simulink model "Appl_DrRestMode_CtrlModel"  (R2018b)
settings: configuration reference "CodeConfig_10_ms" (kept outside this file)
undefined symbols (not defined in the file): D_ClickNapBackPosi, D_ClickNapLengthPosi, D_DRMEM_SPEED_5, D_SoftDistanceDrLegnth, FALSE, TRUE
libraries: DareLib x81, simulink x1
(part 1 of 2)
settings Model: Creator=Administrator  LastModifiedBy=Administrator
settings ConfigSetRef: SourceLocation=Base Workspace

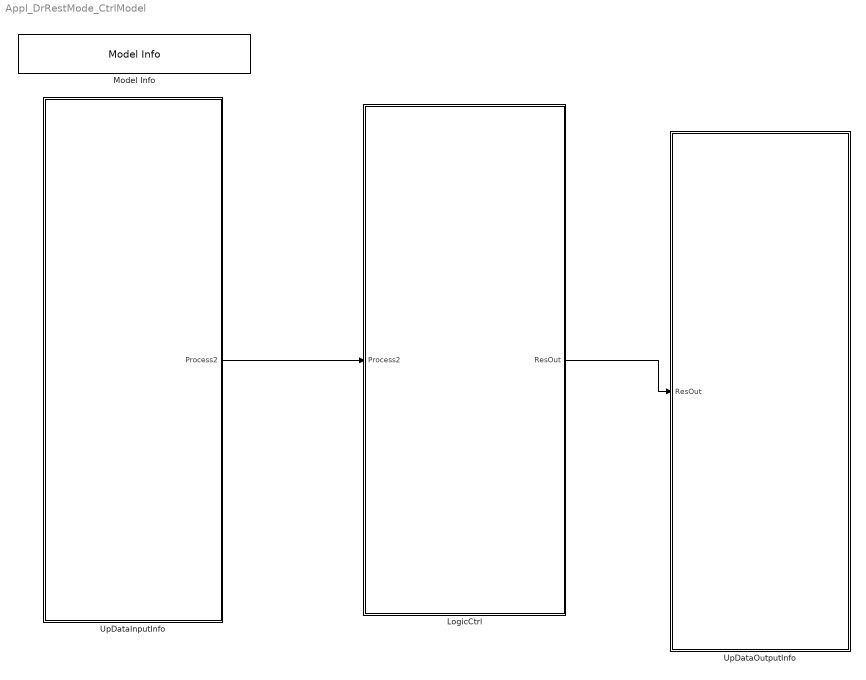
== system Appl_DrRestMode_CtrlModel ==
  LogicCtrl : Subsystem  Priority=2  TreatAsAtomicUnit=on
      settings: RTWSystemCode=Nonreusable function  RTWFcnNameOpts=Use subsystem name
  Model Info : simulink/Model-Wide Utilities/Model Info  Frame=on  DisplayStringWithTags=Version：%<ModelVersion>  HorizontalTextAlignment=Center  LeftAlignmentValue=0.5
  UpDataInputInfo : Subsystem  Priority=1  TreatAsAtomicUnit=on
      settings: RTWSystemCode=Nonreusable function  RTWFcnNameOpts=Use subsystem name
  UpDataOutputInfo : Subsystem  Priority=3  TreatAsAtomicUnit=on
      settings: RTWSystemCode=Nonreusable function  RTWFcnNameOpts=Use subsystem name
  wires:
  LogicCtrl/1(ResOut) -> UpDataOutputInfo/1(ResOut)
  UpDataInputInfo/1(Process2) -> LogicCtrl/1(Process2)

== system Appl_DrRestMode_CtrlModel/LogicCtrl ==
  Process2 : Inport
  Bus Creator : BusCreator  Inputs=13
  Bus Selector : BusSelector  OutputSignals=Res_Stop_Flag.Stop_Flag,Res_Open_Flag.Open_Flag,Res_Close_Flag.Close_Flag,MotorFault_Flag,MassageFault_Flag,DrRestCAll_Ret,Process1.CallHallValue.CallHallVall_Height,Process1.CallHallValue.CallHallVall_Length,Process1.CallHallValue.CallHallVall_Back,Process1.CallHallValue.CallHallVall_Front,Process1.Rte_SignalBus1.DrRes_HeightHallPosi,Process1.Rte_SignalBus1.DrRes_LengthHallPosi,Process1.Rte_SignalBus1.DrRes_BackHallPosi,Process1.Rte_SignalBus1.DrRes_FrontHallPosi,Process1.Rte_SignalBus1.DrRes_AnyoneRelayFaultSts,Process1.Rte_SignalBus1.DrResl_ReCallPosi_Height,Process1.Rte_SignalBus1.DrResl_ReCallPosi_Length,Process1.Rte_SignalBus1.DrResl_ReCallPosi_Back,Process1.Rte_SignalBus1.DrResl_ReCallPosi_Front,Process1.Rte_SignalBus1.DrRes_CurrentMoveType
  ResCtrl : Subsystem  Description=小憩逻辑处理
      settings: AttributesFormatString=%<Description>
  ResOut : Outport
  wires:
  Process2/1 -> Bus Creator/13, Bus Selector/1  "Process2"
  Bus Creator/1 -> ResOut/1  "ResOut"
  ResCtrl/3(DSM_NapMode_FB) -> Bus Creator/3
  ResCtrl/2(DSM_MassageMode_Req) -> Bus Creator/2
  ResCtrl/4(ResCallPosi_Height) -> Bus Creator/4
  ResCtrl/1(DSM_MassageLevel_Req) -> Bus Creator/1
  ResCtrl/5(ResCallPosi_Length) -> Bus Creator/5
  ResCtrl/6(ResCallPosi_Front) -> Bus Creator/6
  ResCtrl/7(ResCallPosi_Back) -> Bus Creator/7
  ResCtrl/8(ResReCallPosi_Back) -> Bus Creator/8
  ResCtrl/9(ResReCallPosi_Front) -> Bus Creator/9
  ResCtrl/10(ResReCallPosi_Height) -> Bus Creator/10
  ResCtrl/11(ResReCallPosi_Length) -> Bus Creator/11
  ResCtrl/12(State_ResDeal) -> Bus Creator/12
  Bus Selector/1 -> ResCtrl/1(Stop_Flag)  "<Stop_Flag>"
  Bus Selector/2 -> ResCtrl/2(Open_Flag)  "<Open_Flag>"
  Bus Selector/3 -> ResCtrl/3(Close_Flag)  "<Close_Flag>"
  Bus Selector/4 -> ResCtrl/4(MotorFault_Flag)  "<MotorFault_Flag>"
  Bus Selector/5 -> ResCtrl/5(MassageFault_Flag)  "<MassageFault_Flag>"
  Bus Selector/6 -> ResCtrl/6(DrRestCAll_Ret)  "<DrRestCAll_Ret>"
  Bus Selector/7 -> ResCtrl/7(CallHallVall_Height)  "<CallHallVall_Height>"
  Bus Selector/8 -> ResCtrl/8(CallHallVall_Length)  "<CallHallVall_Length>"
  Bus Selector/9 -> ResCtrl/9(CallHallVall_Back)  "<CallHallVall_Back>"
  Bus Selector/10 -> ResCtrl/10(CallHallVall_Front)  "<CallHallVall_Front>"
  Bus Selector/11 -> ResCtrl/11(DrRes_HeightHallPosi)  "<DrRes_HeightHallPosi>"
  Bus Selector/12 -> ResCtrl/12(DrRes_LengthHallPosi)  "<DrRes_LengthHallPosi>"
  Bus Selector/13 -> ResCtrl/13(DrRes_BackHallPosi)  "<DrRes_BackHallPosi>"
  Bus Selector/14 -> ResCtrl/14(DrRes_FrontHallPosi)  "<DrRes_FrontHallPosi>"
  Bus Selector/15 -> ResCtrl/15(DrRes_AnyoneRelayFaultSts)  "<DrRes_AnyoneRelayFaultSts>"
  Bus Selector/16 -> ResCtrl/16(DrResl_ReCallPosi_Height)  "<DrResl_ReCallPosi_Height>"
  Bus Selector/17 -> ResCtrl/17(DrResl_ReCallPosi_Length)  "<DrResl_ReCallPosi_Length>"
  Bus Selector/18 -> ResCtrl/18(DrResl_ReCallPosi_Back)  "<DrResl_ReCallPosi_Back>"
  Bus Selector/19 -> ResCtrl/19(DrResl_ReCallPosi_Front)  "<DrResl_ReCallPosi_Front>"
  Bus Selector/20 -> ResCtrl/20(DrRes_CurrentMoveType)  "<DrRes_CurrentMoveType>"

== system Appl_DrRestMode_CtrlModel/UpDataInputInfo ==
  InputSignalProcess1 : Subsystem  Description=预处理1
      settings: AttributesFormatString=%<Description>  RTWSystemCode=Nonreusable function  RTWFcnNameOpts=Use subsystem name
  InputSignalProcess2 : Subsystem  Description=预处理2
      settings: AttributesFormatString=%<Description>  RTWSystemCode=Nonreusable function  RTWFcnNameOpts=Use subsystem name
  RTE : Subsystem  Description=接口自动生成  TreatAsAtomicUnit=on
      settings: AttributesFormatString=%<Description>  RTWSystemCode=Nonreusable function  RTWFcnNameOpts=Use subsystem name
  Process2 : Outport
  wires:
  RTE/1(RTE_Signal) -> InputSignalProcess1/1(Rte_SignalBus)
  InputSignalProcess1/1(Process1) -> InputSignalProcess2/1(Process1)
  InputSignalProcess2/1(Process2) -> Process2/1

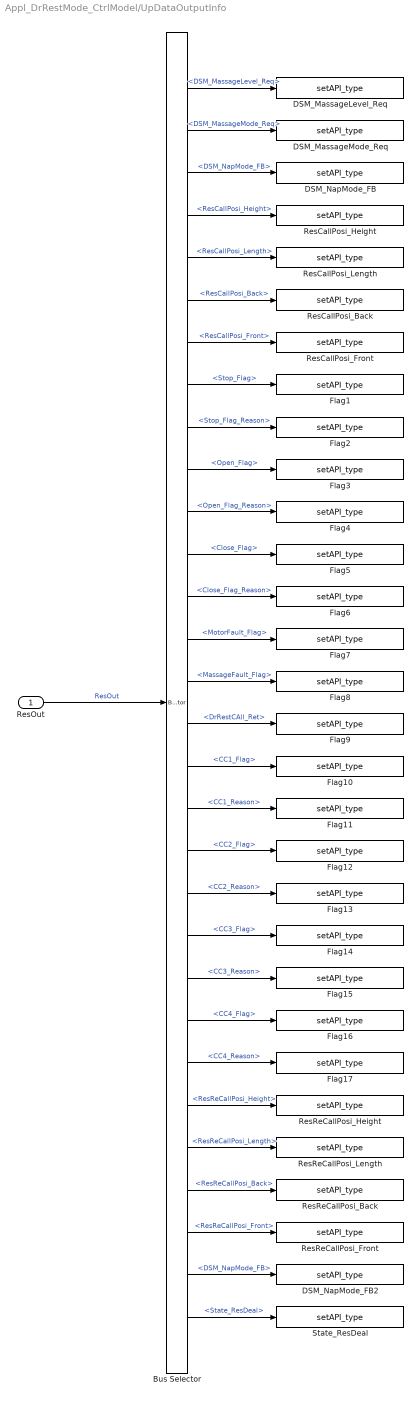
== system Appl_DrRestMode_CtrlModel/UpDataOutputInfo ==
  ResOut : Inport
  Bus Selector : BusSelector  OutputSignals=DSM_MassageLevel_Req,DSM_MassageMode_Req,DSM_NapMode_FB,ResCallPosi_Height,ResCallPosi_Length,ResCallPosi_Back,ResCallPosi_Front,Process2.Res_Stop_Flag.Stop_Flag,Process2.Res_Stop_Flag.Stop_Flag_Reason,Process2.Res_Open_Flag.Open_Flag,Process2.Res_Open_Flag.Open_Flag_Reason,Process2.Res_Close_Flag.Close_Flag,Process2.Res_Close_Flag.Close_Flag_Reason,Process2.MotorFault_Flag,Process2.MassageFault_Flag,Process2.DrRestCAll_Ret,Process2.Process1.CC1.CC1_Flag,Process2.Process1.CC1.CC1_Reason,Process2.Process1.CC2.CC2_Flag,Process2.Process1.CC2.CC2_Reason,Process2.Process1.CC3.CC3_Flag,Process2.Process1.CC3.CC3_Reason,Process2.Process1.CC4.CC4_Flag,Process2.Process1.CC4.CC4_Reason,ResReCallPosi_Height,ResReCallPosi_Length,ResReCallPosi_Back,ResReCallPosi_Front,DSM_NapMode_FB,State_ResDeal
  DSM_MassageLevel_Req : DareLib/Dare/setAPI_type  g_funcname=Rte_SetVfb_Res_MassageLevel_Req  g_param=""  g_type=uint8  g_size=-1
      settings: AttributesFormatString=%<g_funcname>  SourceProductName=Dare Library
  DSM_MassageMode_Req : DareLib/Dare/setAPI_type  g_funcname=Rte_SetVfb_Res_MassageMode_Req  g_param=""  g_type=uint8  g_size=-1
      settings: AttributesFormatString=%<g_funcname>  SourceProductName=Dare Library
  DSM_NapMode_FB : DareLib/Dare/setAPI_type  g_funcname=CanTx_0x3B2_DSM_NapMode_FB  g_param=""  g_type=uint8  g_size=-1
      settings: AttributesFormatString=%<g_funcname>  SourceProductName=Dare Library
  DSM_NapMode_FB2 : DareLib/Dare/setAPI_type  g_funcname=Rte_SetVfb_NapMode  g_param=""  g_type=uint8  g_size=-1
      settings: AttributesFormatString=%<g_funcname>  SourceProductName=Dare Library
  Flag1 : DareLib/Dare/setAPI_type  g_funcname=Rte_SetVfb_Debug_Res_Stop_Flag  g_param=""  g_type=uint8  g_size=-1
      settings: AttributesFormatString=%<g_funcname>  SourceProductName=Dare Library
  Flag10 : DareLib/Dare/setAPI_type  g_funcname=Rte_SetVfb_Debug_Res_CC1_Flag  g_param=""  g_type=uint8  g_size=-1
      settings: AttributesFormatString=%<g_funcname>  SourceProductName=Dare Library
  Flag11 : DareLib/Dare/setAPI_type  g_funcname=Rte_SetVfb_Debug_Res_CC1_Reason  g_param=""  g_type=uint8  g_size=-1
      settings: AttributesFormatString=%<g_funcname>  SourceProductName=Dare Library
  Flag12 : DareLib/Dare/setAPI_type  g_funcname=Rte_SetVfb_Debug_Res_CC2_Flag  g_param=""  g_type=uint8  g_size=-1
      settings: AttributesFormatString=%<g_funcname>  SourceProductName=Dare Library
  Flag13 : DareLib/Dare/setAPI_type  g_funcname=Rte_SetVfb_Debug_Res_CC2_Reason  g_param=""  g_type=uint8  g_size=-1
      settings: AttributesFormatString=%<g_funcname>  SourceProductName=Dare Library
  Flag14 : DareLib/Dare/setAPI_type  g_funcname=Rte_SetVfb_Debug_Res_CC3_Flag  g_param=""  g_type=uint8  g_size=-1
      settings: AttributesFormatString=%<g_funcname>  SourceProductName=Dare Library
  Flag15 : DareLib/Dare/setAPI_type  g_funcname=Rte_SetVfb_Debug_Res_CC3_Reason  g_param=""  g_type=uint8  g_size=-1
      settings: AttributesFormatString=%<g_funcname>  SourceProductName=Dare Library
  Flag16 : DareLib/Dare/setAPI_type  g_funcname=Rte_SetVfb_Debug_Res_CC4_Flag  g_param=""  g_type=uint8  g_size=-1
      settings: AttributesFormatString=%<g_funcname>  SourceProductName=Dare Library
  Flag17 : DareLib/Dare/setAPI_type  g_funcname=Rte_SetVfb_Debug_Res_CC4_Reason  g_param=""  g_type=uint8  g_size=-1
      settings: AttributesFormatString=%<g_funcname>  SourceProductName=Dare Library
  Flag2 : DareLib/Dare/setAPI_type  g_funcname=Rte_SetVfb_Debug_Res_Stop_Flag_Reason  g_param=""  g_type=uint8  g_size=-1
      settings: AttributesFormatString=%<g_funcname>  SourceProductName=Dare Library
  Flag3 : DareLib/Dare/setAPI_type  g_funcname=Rte_SetVfb_Debug_Res_Open_Flag  g_param=""  g_type=uint8  g_size=-1
      settings: AttributesFormatString=%<g_funcname>  SourceProductName=Dare Library
  Flag4 : DareLib/Dare/setAPI_type  g_funcname=Rte_SetVfb_Debug_Res_Open_Flag_Reason  g_param=""  g_type=uint8  g_size=-1
      settings: AttributesFormatString=%<g_funcname>  SourceProductName=Dare Library
  Flag5 : DareLib/Dare/setAPI_type  g_funcname=Rte_SetVfb_Debug_Res_Colse_Flag  g_param=""  g_type=uint8  g_size=-1
      settings: AttributesFormatString=%<g_funcname>  SourceProductName=Dare Library
  Flag6 : DareLib/Dare/setAPI_type  g_funcname=Rte_SetVfb_Debug_Res_Colse_Flag_Reason  g_param=""  g_type=uint8  g_size=-1
      settings: AttributesFormatString=%<g_funcname>  SourceProductName=Dare Library
  Flag7 : DareLib/Dare/setAPI_type  g_funcname=Rte_SetVfb_Debug_Res_MotroFault_Flag  g_param=""  g_type=uint8  g_size=-1
      settings: AttributesFormatString=%<g_funcname>  SourceProductName=Dare Library
  Flag8 : DareLib/Dare/setAPI_type  g_funcname=Rte_SetVfb_Debug_Res_MassageFault_Flag  g_param=""  g_type=uint8  g_size=-1
      settings: AttributesFormatString=%<g_funcname>  SourceProductName=Dare Library
  Flag9 : DareLib/Dare/setAPI_type  g_funcname=Rte_SetVfb_Debug_Res_DrRestCAllRet  g_param=""  g_type=uint8  g_size=-1
      settings: AttributesFormatString=%<g_funcname>  SourceProductName=Dare Library
  ResCallPosi_Back : DareLib/Dare/setAPI_type  g_funcname=Rte_SetVfb_DrResBackReqPosi  g_param=""  g_type=uint16  g_size=-1
      settings: AttributesFormatString=%<g_funcname>  SourceProductName=Dare Library
  ResCallPosi_Front : DareLib/Dare/setAPI_type  g_funcname=Rte_SetVfb_DrResFrontReqPosi  g_param=""  g_type=uint16  g_size=-1
      settings: AttributesFormatString=%<g_funcname>  SourceProductName=Dare Library
  ResCallPosi_Height : DareLib/Dare/setAPI_type  g_funcname=Rte_SetVfb_DrResHeightReqPosi  g_param=""  g_type=uint16  g_size=-1
      settings: AttributesFormatString=%<g_funcname>  SourceProductName=Dare Library
  ResCallPosi_Length : DareLib/Dare/setAPI_type  g_funcname=Rte_SetVfb_DrResLengthReqPosi  g_param=""  g_type=uint16  g_size=-1
      settings: AttributesFormatString=%<g_funcname>  SourceProductName=Dare Library
  ResReCallPosi_Back : DareLib/Dare/setAPI_type  g_funcname=Rte_SetVfb_DrResBackReCallPosi  g_param=""  g_type=uint16  g_size=-1
      settings: AttributesFormatString=%<g_funcname>  SourceProductName=Dare Library
  ResReCallPosi_Front : DareLib/Dare/setAPI_type  g_funcname=Rte_SetVfb_DrResFrontReCallPosi  g_param=""  g_type=uint16  g_size=-1
      settings: AttributesFormatString=%<g_funcname>  SourceProductName=Dare Library
  ResReCallPosi_Height : DareLib/Dare/setAPI_type  g_funcname=Rte_SetVfb_DrResHeightReCallPosi  g_param=""  g_type=uint16  g_size=-1
      settings: AttributesFormatString=%<g_funcname>  SourceProductName=Dare Library
  ResReCallPosi_Length : DareLib/Dare/setAPI_type  g_funcname=Rte_SetVfb_DrResLengthReCallPosi  g_param=""  g_type=uint16  g_size=-1
      settings: AttributesFormatString=%<g_funcname>  SourceProductName=Dare Library
  State_ResDeal : DareLib/Dare/setAPI_type  g_funcname=Rte_SetVfb_Debug_Res_State_ResDeal  g_param=""  g_type=uint8  g_size=-1
      settings: AttributesFormatString=%<g_funcname>  SourceProductName=Dare Library
  wires:
  ResOut/1 -> Bus Selector/1  "ResOut"
  Bus Selector/30 -> State_ResDeal/1  "<State_ResDeal>"
  Bus Selector/29 -> DSM_NapMode_FB2/1  "<DSM_NapMode_FB>"
  Bus Selector/28 -> ResReCallPosi_Front/1  "<ResReCallPosi_Front>"
  Bus Selector/27 -> ResReCallPosi_Back/1  "<ResReCallPosi_Back>"
  Bus Selector/26 -> ResReCallPosi_Length/1  "<ResReCallPosi_Length>"
  Bus Selector/25 -> ResReCallPosi_Height/1  "<ResReCallPosi_Height>"
  Bus Selector/24 -> Flag17/1  "<CC4_Reason>"
  Bus Selector/23 -> Flag16/1  "<CC4_Flag>"
  Bus Selector/22 -> Flag15/1  "<CC3_Reason>"
  Bus Selector/21 -> Flag14/1  "<CC3_Flag>"
  Bus Selector/20 -> Flag13/1  "<CC2_Reason>"
  Bus Selector/19 -> Flag12/1  "<CC2_Flag>"
  Bus Selector/18 -> Flag11/1  "<CC1_Reason>"
  Bus Selector/17 -> Flag10/1  "<CC1_Flag>"
  Bus Selector/16 -> Flag9/1  "<DrRestCAll_Ret>"
  Bus Selector/15 -> Flag8/1  "<MassageFault_Flag>"
  Bus Selector/14 -> Flag7/1  "<MotorFault_Flag>"
  Bus Selector/13 -> Flag6/1  "<Close_Flag_Reason>"
  Bus Selector/12 -> Flag5/1  "<Close_Flag>"
  Bus Selector/11 -> Flag4/1  "<Open_Flag_Reason>"
  Bus Selector/10 -> Flag3/1  "<Open_Flag>"
  Bus Selector/9 -> Flag2/1  "<Stop_Flag_Reason>"
  Bus Selector/8 -> Flag1/1  "<Stop_Flag>"
  Bus Selector/7 -> ResCallPosi_Front/1  "<ResCallPosi_Front>"
  Bus Selector/6 -> ResCallPosi_Back/1  "<ResCallPosi_Back>"
  Bus Selector/5 -> ResCallPosi_Length/1  "<ResCallPosi_Length>"
  Bus Selector/4 -> ResCallPosi_Height/1  "<ResCallPosi_Height>"
  Bus Selector/3 -> DSM_NapMode_FB/1  "<DSM_NapMode_FB>"
  Bus Selector/2 -> DSM_MassageMode_Req/1  "<DSM_MassageMode_Req>"
  Bus Selector/1 -> DSM_MassageLevel_Req/1  "<DSM_MassageLevel_Req>"

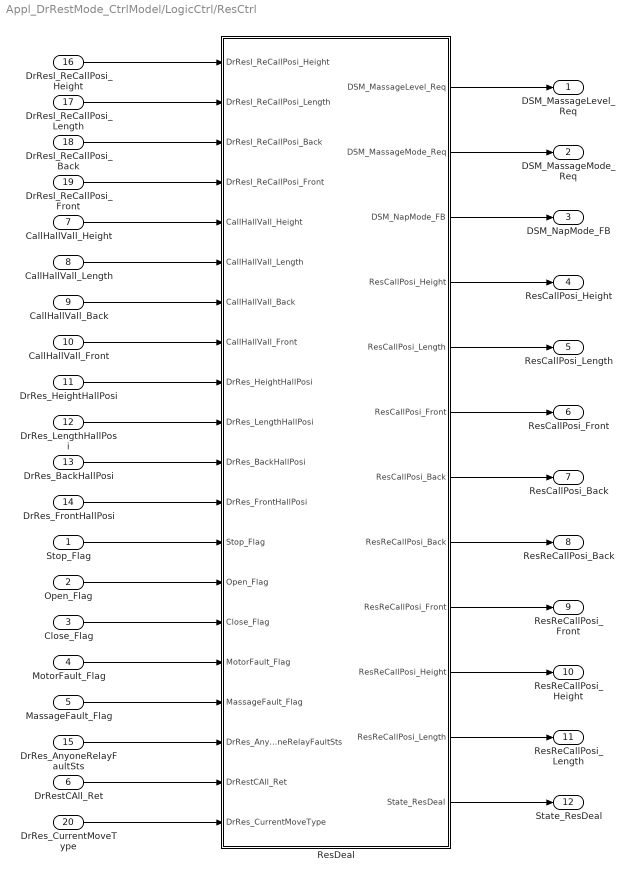
== system Appl_DrRestMode_CtrlModel/LogicCtrl/ResCtrl ==
  Stop_Flag : Inport
  Open_Flag : Inport  Port=2
  Close_Flag : Inport  Port=3
  MotorFault_Flag : Inport  Port=4
  MassageFault_Flag : Inport  Port=5
  DrRestCAll_Ret : Inport  Port=6
  CallHallVall_Height : Inport  Port=7
  CallHallVall_Length : Inport  Port=8
  CallHallVall_Back : Inport  Port=9
  CallHallVall_Front : Inport  Port=10
  DrRes_HeightHallPosi : Inport  Port=11
  DrRes_LengthHallPosi : Inport  Port=12
  DrRes_BackHallPosi : Inport  Port=13
  DrRes_FrontHallPosi : Inport  Port=14
  DrRes_AnyoneRelayFaultSts : Inport  Port=15
  DrResl_ReCallPosi_Height : Inport  Port=16
  DrResl_ReCallPosi_Length : Inport  Port=17
  DrResl_ReCallPosi_Back : Inport  Port=18
  DrResl_ReCallPosi_Front : Inport  Port=19
  DrRes_CurrentMoveType : Inport  Port=20
  ResDeal : Stateflow chart  TreatAsAtomicUnit=on
  DSM_MassageLevel_Req : Outport
  DSM_MassageMode_Req : Outport  Port=2
  DSM_NapMode_FB : Outport  Port=3
  ResCallPosi_Height : Outport  Port=4
  ResCallPosi_Length : Outport  Port=5
  ResCallPosi_Front : Outport  Port=6
  ResCallPosi_Back : Outport  Port=7
  ResReCallPosi_Back : Outport  Port=8
  ResReCallPosi_Front : Outport  Port=9
  ResReCallPosi_Height : Outport  Port=10
  ResReCallPosi_Length : Outport  Port=11
  State_ResDeal : Outport  Port=12
  wires:
  ResDeal/1(DSM_MassageLevel_Req) -> DSM_MassageLevel_Req/1
  ResDeal/2(DSM_MassageMode_Req) -> DSM_MassageMode_Req/1
  ResDeal/3(DSM_NapMode_FB) -> DSM_NapMode_FB/1
  ResDeal/7(ResCallPosi_Back) -> ResCallPosi_Back/1
  ResDeal/6(ResCallPosi_Front) -> ResCallPosi_Front/1
  ResDeal/5(ResCallPosi_Length) -> ResCallPosi_Length/1
  ResDeal/4(ResCallPosi_Height) -> ResCallPosi_Height/1
  ResDeal/8(ResReCallPosi_Back) -> ResReCallPosi_Back/1
  ResDeal/9(ResReCallPosi_Front) -> ResReCallPosi_Front/1
  ResDeal/10(ResReCallPosi_Height) -> ResReCallPosi_Height/1
  ResDeal/11(ResReCallPosi_Length) -> ResReCallPosi_Length/1
  ResDeal/12(State_ResDeal) -> State_ResDeal/1
  CallHallVall_Height/1 -> ResDeal/5(CallHallVall_Height)
  DrResl_ReCallPosi_Height/1 -> ResDeal/1(DrResl_ReCallPosi_Height)
  DrResl_ReCallPosi_Length/1 -> ResDeal/2(DrResl_ReCallPosi_Length)
  DrResl_ReCallPosi_Back/1 -> ResDeal/3(DrResl_ReCallPosi_Back)
  DrResl_ReCallPosi_Front/1 -> ResDeal/4(DrResl_ReCallPosi_Front)
  CallHallVall_Length/1 -> ResDeal/6(CallHallVall_Length)
  DrRes_HeightHallPosi/1 -> ResDeal/9(DrRes_HeightHallPosi)
  DrRes_LengthHallPosi/1 -> ResDeal/10(DrRes_LengthHallPosi)
  DrRes_BackHallPosi/1 -> ResDeal/11(DrRes_BackHallPosi)
  DrRes_FrontHallPosi/1 -> ResDeal/12(DrRes_FrontHallPosi)
  Stop_Flag/1 -> ResDeal/13(Stop_Flag)
  Open_Flag/1 -> ResDeal/14(Open_Flag)
  CallHallVall_Back/1 -> ResDeal/7(CallHallVall_Back)
  CallHallVall_Front/1 -> ResDeal/8(CallHallVall_Front)
  MassageFault_Flag/1 -> ResDeal/17(MassageFault_Flag)
  Close_Flag/1 -> ResDeal/15(Close_Flag)
  MotorFault_Flag/1 -> ResDeal/16(MotorFault_Flag)
  DrRes_AnyoneRelayFaultSts/1 -> ResDeal/18(DrRes_AnyoneRelayFaultSts)
  DrRestCAll_Ret/1 -> ResDeal/19(DrRestCAll_Ret)
  DrRes_CurrentMoveType/1 -> ResDeal/20(DrRes_CurrentMoveType)

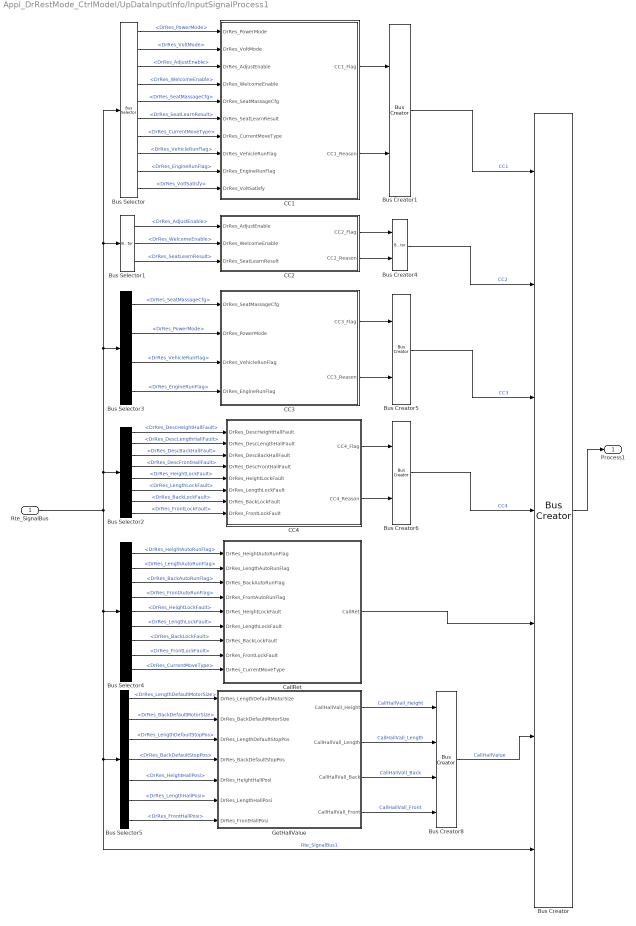
== system Appl_DrRestMode_CtrlModel/UpDataInputInfo/InputSignalProcess1 ==
  Rte_SignalBus : Inport
  Bus Creator : BusCreator  Inputs=7
  Bus Creator{1,4..6} (4 alike) : BusCreator  Inputs=2
  Bus Creator8 : BusCreator  Inputs=4
  Bus Selector : BusSelector  OutputSignals=DrRes_PowerMode,DrRes_VoltMode,DrRes_AdjustEnable,DrRes_WelcomeEnable,DrRes_SeatMassageCfg,DrRes_SeatLearnResult,DrRes_CurrentMoveType,DrRes_VehicleRunFlag,DrRes_EngineRunFlag,DrRes_VoltSatisfy
  Bus Selector1 : BusSelector  OutputSignals=DrRes_AdjustEnable,DrRes_WelcomeEnable,DrRes_SeatLearnResult
  Bus Selector2 : BusSelector  OutputSignals=DrRes_DescHeightHallFault,DrRes_DescLengthHallFault,DrRes_DescBackHallFault,DrRes_DescFrontHallFault,DrRes_HeightLockFault,DrRes_LengthLockFault,DrRes_BackLockFault,DrRes_FrontLockFault
  Bus Selector3 : BusSelector  OutputSignals=DrRes_SeatMassageCfg,DrRes_PowerMode,DrRes_VehicleRunFlag,DrRes_EngineRunFlag
  Bus Selector4 : BusSelector  OutputSignals=DrRes_HeightAutoRunFlag,DrRes_LengthAutoRunFlag,DrRes_BackAutoRunFlag,DrRes_FrontAutoRunFlag,DrRes_HeightLockFault,DrRes_LengthLockFault,DrRes_BackLockFault,DrRes_FrontLockFault,DrRes_CurrentMoveType
  Bus Selector5 : BusSelector  OutputSignals=DrRes_LengthDefaultMotorSize,DrRes_BackDefaultMotorSize,DrRes_LengthDefaultStopPos,DrRes_BackDefaultStopPos,DrRes_HeightHallPosi,DrRes_LengthHallPosi,DrRes_FrontHallPosi
  CC1 : Subsystem
      settings: AttributesFormatString=%<Description>
  CC2 : Subsystem
      settings: AttributesFormatString=%<Description>
  CC3 : Subsystem
      settings: AttributesFormatString=%<Description>
  CC4 : Subsystem
      settings: AttributesFormatString=%<Description>
  CallRet : Subsystem  Description=坐标调用结果
      settings: AttributesFormatString=%<Description>
  GetHallValue : Subsystem  Description=获取小憩开启的坐标值
      settings: AttributesFormatString=%<Description>
  Process1 : Outport
  wires:
  Bus Creator/1 -> Process1/1
  Rte_SignalBus/1 -> Bus Selector3/1, Bus Selector/1, Bus Selector1/1, Bus Selector2/1, Bus Creator/7, Bus Selector5/1, Bus Selector4/1  "Rte_SignalBus1"
  Bus Creator1/1 -> Bus Creator/1  "CC1"
  Bus Selector1/1 -> CC2/1(DrRes_AdjustEnable)  "<DrRes_AdjustEnable>"
  Bus Selector1/2 -> CC2/2(DrRes_WelcomeEnable)  "<DrRes_WelcomeEnable>"
  Bus Selector1/3 -> CC2/3(DrRes_SeatLearnResult)  "<DrRes_SeatLearnResult>"
  Bus Selector2/1 -> CC4/1(DrRes_DescHeightHallFault)  "<DrRes_DescHeightHallFault>"
  Bus Selector4/1 -> CallRet/1(DrRes_HeightAutoRunFlag)  "<DrRes_HeightAutoRunFlag>"
  Bus Selector4/2 -> CallRet/2(DrRes_LengthAutoRunFlag)  "<DrRes_LengthAutoRunFlag>"
  Bus Selector4/3 -> CallRet/3(DrRes_BackAutoRunFlag)  "<DrRes_BackAutoRunFlag>"
  Bus Selector4/4 -> CallRet/4(DrRes_FrontAutoRunFlag)  "<DrRes_FrontAutoRunFlag>"
  Bus Selector4/5 -> CallRet/5(DrRes_HeightLockFault)  "<DrRes_HeightLockFault>"
  Bus Selector4/6 -> CallRet/6(DrRes_LengthLockFault)  "<DrRes_LengthLockFault>"
  Bus Selector4/7 -> CallRet/7(DrRes_BackLockFault)  "<DrRes_BackLockFault>"
  Bus Selector4/8 -> CallRet/8(DrRes_FrontLockFault)  "<DrRes_FrontLockFault>"
  CC4/1("CC4_Flag ") -> Bus Creator6/1
  CC4/2(CC4_Reason) -> Bus Creator6/2
  CC1/1("CC1_Flag ") -> Bus Creator1/1
  CC1/2(CC1_Reason) -> Bus Creator1/2
  CC2/1("CC2_Flag ") -> Bus Creator4/1
  CC2/2(CC2_Reason) -> Bus Creator4/2
  CC3/1("CC3_Flag ") -> Bus Creator5/1
  CC3/2(CC3_Reason) -> Bus Creator5/2
  Bus Creator4/1 -> Bus Creator/2  "CC2"
  Bus Creator5/1 -> Bus Creator/3  "CC3"
  Bus Creator6/1 -> Bus Creator/4  "CC4"
  CallRet/1(CallRet) -> Bus Creator/5
  Bus Creator8/1 -> Bus Creator/6  "CallHallValue"
  GetHallValue/1(CallHallVall_Height) -> Bus Creator8/1  "CallHallVall_Height"
  GetHallValue/2(CallHallVall_Length) -> Bus Creator8/2  "CallHallVall_Length"
  GetHallValue/3(CallHallVall_Back) -> Bus Creator8/3  "CallHallVall_Back"
  GetHallValue/4(CallHallVall_Front) -> Bus Creator8/4  "CallHallVall_Front"
  Bus Selector4/9 -> CallRet/9(DrRes_CurrentMoveType)  "<DrRes_CurrentMoveType>"
  Bus Selector/1 -> CC1/1(DrRes_PowerMode)  "<DrRes_PowerMode>"
  Bus Selector/2 -> CC1/2(DrRes_VoltMode)  "<DrRes_VoltMode>"
  Bus Selector/3 -> CC1/3(DrRes_AdjustEnable)  "<DrRes_AdjustEnable>"
  Bus Selector/4 -> CC1/4(DrRes_WelcomeEnable)  "<DrRes_WelcomeEnable>"
  Bus Selector/5 -> CC1/5(DrRes_SeatMassageCfg)  "<DrRes_SeatMassageCfg>"
  Bus Selector/6 -> CC1/6(DrRes_SeatLearnResult)  "<DrRes_SeatLearnResult>"
  Bus Selector/7 -> CC1/7(DrRes_CurrentMoveType)  "<DrRes_CurrentMoveType>"
  Bus Selector/8 -> CC1/8(DrRes_VehicleRunFlag)  "<DrRes_VehicleRunFlag>"
  Bus Selector/9 -> CC1/9(DrRes_EngineRunFlag)  "<DrRes_EngineRunFlag>"
  Bus Selector3/1 -> CC3/1(DrRes_SeatMassageCfg)  "<DrRes_SeatMassageCfg>"
  Bus Selector3/2 -> CC3/2(DrRes_PowerMode)  "<DrRes_PowerMode>"
  Bus Selector3/3 -> CC3/3(DrRes_VehicleRunFlag)  "<DrRes_VehicleRunFlag>"
  Bus Selector3/4 -> CC3/4(DrRes_EngineRunFlag)  "<DrRes_EngineRunFlag>"
  Bus Selector/10 -> CC1/10(DrRes_VoltSatisfy)  "<DrRes_VoltSatisfy>"
  Bus Selector5/1 -> GetHallValue/1(DrRes_LengthDefaultMotorSize)  "<DrRes_LengthDefaultMotorSize>"
  Bus Selector5/2 -> GetHallValue/2(DrRes_BackDefaultMotorSize)  "<DrRes_BackDefaultMotorSize>"
  Bus Selector5/3 -> GetHallValue/3(DrRes_LengthDefaultStopPos)  "<DrRes_LengthDefaultStopPos>"
  Bus Selector5/4 -> GetHallValue/4(DrRes_BackDefaultStopPos)  "<DrRes_BackDefaultStopPos>"
  Bus Selector5/5 -> GetHallValue/5(DrRes_HeightHallPosi)  "<DrRes_HeightHallPosi>"
  Bus Selector5/6 -> GetHallValue/6(DrRes_LengthHallPosi)  "<DrRes_LengthHallPosi>"
  Bus Selector5/7 -> GetHallValue/7(DrRes_FrontHallPosi)  "<DrRes_FrontHallPosi>"
  Bus Selector2/3 -> CC4/3(DrRes_DescBackHallFault)  "<DrRes_DescBackHallFault>"
  Bus Selector2/4 -> CC4/4(DrRes_DescFrontHallFault)  "<DrRes_DescFrontHallFault>"
  Bus Selector2/2 -> CC4/2(DrRes_DescLengthHallFault)  "<DrRes_DescLengthHallFault>"
  Bus Selector2/5 -> CC4/5(DrRes_HeightLockFault)  "<DrRes_HeightLockFault>"
  Bus Selector2/6 -> CC4/6(DrRes_LengthLockFault)  "<DrRes_LengthLockFault>"
  Bus Selector2/7 -> CC4/7(DrRes_BackLockFault)  "<DrRes_BackLockFault>"
  Bus Selector2/8 -> CC4/8(DrRes_FrontLockFault)  "<DrRes_FrontLockFault>"

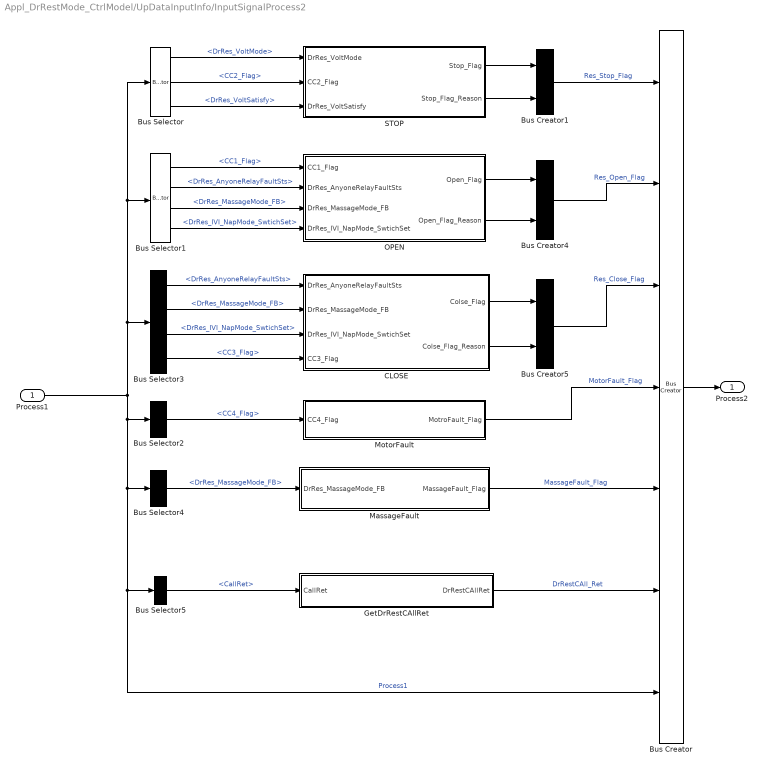
== system Appl_DrRestMode_CtrlModel/UpDataInputInfo/InputSignalProcess2 ==
  Process1 : Inport
  Bus Creator : BusCreator  Inputs=7
  Bus Creator1 : BusCreator  Inputs=2
  Bus Creator4 : BusCreator  Inputs=2
  Bus Creator5 : BusCreator  Inputs=2
  Bus Selector : BusSelector  OutputSignals=Rte_SignalBus1.DrRes_VoltMode,CC2.CC2_Flag,Rte_SignalBus1.DrRes_VoltSatisfy
  Bus Selector1 : BusSelector  OutputSignals=CC1.CC1_Flag,Rte_SignalBus1.DrRes_AnyoneRelayFaultSts,Rte_SignalBus1.DrRes_MassageMode_FB,Rte_SignalBus1.DrRes_IVI_NapMode_SwtichSet
  Bus Selector2 : BusSelector  OutputSignals=CC4.CC4_Flag
  Bus Selector3 : BusSelector  OutputSignals=Rte_SignalBus1.DrRes_AnyoneRelayFaultSts,Rte_SignalBus1.DrRes_MassageMode_FB,Rte_SignalBus1.DrRes_IVI_NapMode_SwtichSet,CC3.CC3_Flag
  Bus Selector4 : BusSelector  OutputSignals=Rte_SignalBus1.DrRes_MassageMode_FB
  Bus Selector5 : BusSelector  OutputSignals=CallRet
  CLOSE : Subsystem  Description=小憩关闭请求标志
      settings: AttributesFormatString=%<Description>
  GetDrRestCAllRet : Subsystem  Description=小憩调用结果
      settings: AttributesFormatString=%<Description>
  MassageFault : Subsystem  Description=按摩故障标志位
      settings: AttributesFormatString=%<Description>
  MotorFault : Subsystem  Description=电机故障标志位
      settings: AttributesFormatString=%<Description>
  OPEN : Subsystem  Description=小憩开启请求标志
      settings: AttributesFormatString=%<Description>
  STOP : Subsystem  Description=小憩停止动作标志位
      settings: AttributesFormatString=%<Description>
  Process2 : Outport
  wires:
  Bus Creator5/1 -> Bus Creator/3  "Res_Close_Flag"
  Bus Creator4/1 -> Bus Creator/2  "Res_Open_Flag"
  CLOSE/2(Colse_Flag_Reason) -> Bus Creator5/2
  CLOSE/1("Colse_Flag ") -> Bus Creator5/1
  OPEN/2(Open_Flag_Reason) -> Bus Creator4/2
  OPEN/1("Open_Flag ") -> Bus Creator4/1
  STOP/2(Stop_Flag_Reason) -> Bus Creator1/2
  STOP/1("Stop_Flag ") -> Bus Creator1/1
  MotorFault/1("MotroFault_Flag ") -> Bus Creator/4  "MotorFault_Flag"
  Bus Selector2/1 -> MotorFault/1(CC4_Flag)  "<CC4_Flag>"
  Bus Creator1/1 -> Bus Creator/1  "Res_Stop_Flag"
  Process1/1 -> Bus Creator/7, Bus Selector5/1, Bus Selector4/1, Bus Selector2/1, Bus Selector1/1, Bus Selector/1, Bus Selector3/1  "Process1"
  Bus Creator/1 -> Process2/1
  Bus Selector/2 -> STOP/2(CC2_Flag)  "<CC2_Flag>"
  Bus Selector/1 -> STOP/1(DrRes_VoltMode)  "<DrRes_VoltMode>"
  Bus Selector1/1 -> OPEN/1(CC1_Flag)  "<CC1_Flag>"
  Bus Selector1/2 -> OPEN/2(DrRes_AnyoneRelayFaultSts)  "<DrRes_AnyoneRelayFaultSts>"
  Bus Selector1/3 -> OPEN/3(DrRes_MassageMode_FB)  "<DrRes_MassageMode_FB>"
  Bus Selector1/4 -> OPEN/4(DrRes_IVI_NapMode_SwtichSet)  "<DrRes_IVI_NapMode_SwtichSet>"
  Bus Selector3/1 -> CLOSE/1(DrRes_AnyoneRelayFaultSts)  "<DrRes_AnyoneRelayFaultSts>"
  Bus Selector3/2 -> CLOSE/2(DrRes_MassageMode_FB)  "<DrRes_MassageMode_FB>"
  Bus Selector3/3 -> CLOSE/3(DrRes_IVI_NapMode_SwtichSet)  "<DrRes_IVI_NapMode_SwtichSet>"
  Bus Selector3/4 -> CLOSE/4(CC3_Flag)  "<CC3_Flag>"
  Bus Selector4/1 -> MassageFault/1(DrRes_MassageMode_FB)  "<DrRes_MassageMode_FB>"
  Bus Selector5/1 -> GetDrRestCAllRet/1(CallRet)  "<CallRet>"
  GetDrRestCAllRet/1(DrRestCAllRet) -> Bus Creator/6  "DrRestCAll_Ret"
  MassageFault/1("MassageFault_Flag ") -> Bus Creator/5  "MassageFault_Flag"
  Bus Selector/3 -> STOP/3(DrRes_VoltSatisfy)  "<DrRes_VoltSatisfy>"

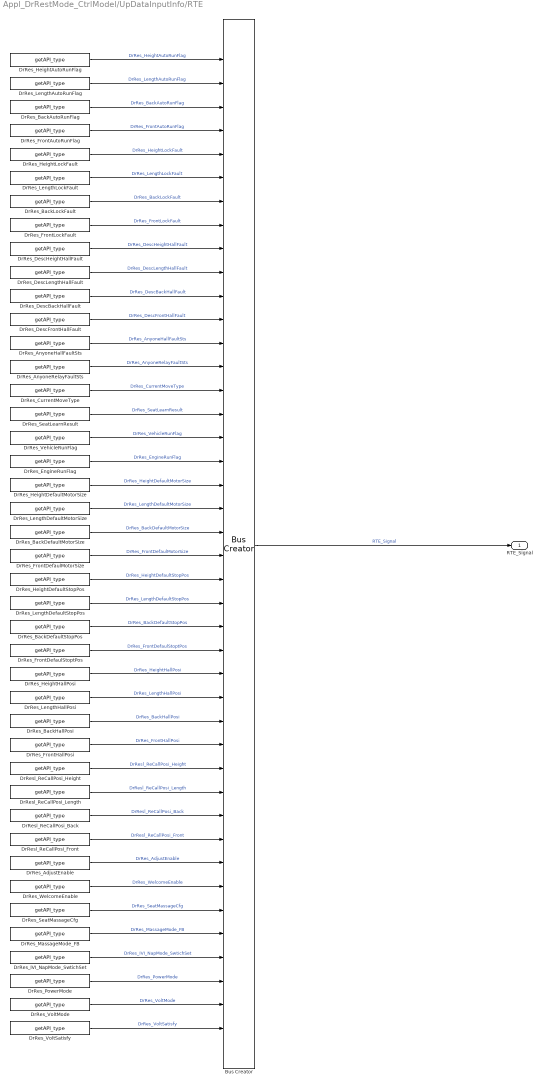
== system Appl_DrRestMode_CtrlModel/UpDataInputInfo/RTE ==
  Bus Creator : BusCreator  Inputs=42
  DrRes_AdjustEnable : DareLib/Dare/getAPI_type  g_funcname=Srvl_GetMemIndexDataU8  g_param=EN_MemIndex_DrAdjustConfig  g_type=uint8  g_size=-1
      settings: AttributesFormatString=%<g_funcname>  SourceProductName=Dare Library
  DrRes_AnyoneHallFaultSts : DareLib/Dare/getAPI_type  g_funcname=Rte_GetVfb_DrAnyoneHallErr  g_param=""  g_type=uint8  g_size=-1
      settings: AttributesFormatString=%<g_funcname>  SourceProductName=Dare Library
  DrRes_AnyoneRelayFaultSts : DareLib/Dare/getAPI_type  g_funcname=Rte_GetVfb_DrAnyoneRelayAdheErr  g_param=""  g_type=uint8  g_size=-1
      settings: AttributesFormatString=%<g_funcname>  SourceProductName=Dare Library
  DrRes_BackAutoRunFlag : DareLib/Dare/getAPI_type  g_funcname=Rte_GetVfb_DrBackAutoRunFlag  g_param=""  g_type=uint8  g_enum=enSeatAutoRunSts  g_size=-1
      settings: AttributesFormatString=%<g_funcname>  SourceProductName=Dare Library
  DrRes_BackDefaultMotorSize : DareLib/Dare/getAPI_type  g_funcname=Cdd_GetMotorSize  g_param=EN_DriverBack  g_type=uint16  g_size=-1
      settings: AttributesFormatString=%<g_funcname>  SourceProductName=Dare Library
  DrRes_BackDefaultStopPos : DareLib/Dare/getAPI_type  g_funcname=Cdd_GetMotorHardStop  g_param=EN_DriverBack  g_type=uint16  g_size=-1
      settings: AttributesFormatString=%<g_funcname>  SourceProductName=Dare Library
  DrRes_BackHallPosi : DareLib/Dare/getAPI_type  g_funcname=Cdd_GetCurrentHallCnt  g_param=EN_DriverBack  g_type=uint16  g_size=-1
      settings: AttributesFormatString=%<g_funcname>  SourceProductName=Dare Library
  DrRes_BackLockFault : DareLib/Dare/getAPI_type  g_funcname=Rte_GetVfb_DrBackStallErr  g_param=""  g_type=uint8  g_size=-1
      settings: AttributesFormatString=%<g_funcname>  SourceProductName=Dare Library
  DrRes_CurrentMoveType : DareLib/Dare/getAPI_type  g_funcname=Rte_GetVfb_DrMoveType  g_param=""  g_type=uint8  g_enum=enSeatMotorRunType  g_size=-1
      settings: AttributesFormatString=%<g_funcname>  SourceProductName=Dare Library
  DrRes_DescBackHallFault : DareLib/Dare/getAPI_type  g_funcname=Rte_GetVfb_DrBackHallErr  g_param=""  g_type=uint8  g_size=-1
      settings: AttributesFormatString=%<g_funcname>  SourceProductName=Dare Library
  DrRes_DescFrontHallFault : DareLib/Dare/getAPI_type  g_funcname=Rte_GetVfb_DrFrontHallErr  g_param=""  g_type=uint8  g_size=-1
      settings: AttributesFormatString=%<g_funcname>  SourceProductName=Dare Library
  DrRes_DescHeightHallFault : DareLib/Dare/getAPI_type  g_funcname=Rte_GetVfb_DrHeightHallErr  g_param=""  g_type=uint8  g_size=-1
      settings: AttributesFormatString=%<g_funcname>  SourceProductName=Dare Library
  DrRes_DescLengthHallFault : DareLib/Dare/getAPI_type  g_funcname=Rte_GetVfb_DrLengthHallErr  g_param=""  g_type=uint8  g_size=-1
      settings: AttributesFormatString=%<g_funcname>  SourceProductName=Dare Library
  DrRes_EngineRunFlag : DareLib/Dare/getAPI_type  g_funcname=Rte_GetVfb_EngineRunFlag  g_param=""  g_type=uint8  g_size=-1
      settings: AttributesFormatString=%<g_funcname>  SourceProductName=Dare Library
  DrRes_FrontAutoRunFlag : DareLib/Dare/getAPI_type  g_funcname=Rte_GetVfb_DrFrontAutoRunFlag  g_param=""  g_type=uint8  g_enum=enSeatAutoRunSts  g_size=-1
      settings: AttributesFormatString=%<g_funcname>  SourceProductName=Dare Library
  DrRes_FrontDefaulMotorSize : DareLib/Dare/getAPI_type  g_funcname=Cdd_GetMotorSize  g_param=EN_DriverFront  g_type=uint16  g_size=-1
      settings: AttributesFormatString=%<g_funcname>  SourceProductName=Dare Library
  DrRes_FrontDefaulStoptPos : DareLib/Dare/getAPI_type  g_funcname=Cdd_GetMotorHardStop  g_param=EN_DriverFront  g_type=uint16  g_size=-1
      settings: AttributesFormatString=%<g_funcname>  SourceProductName=Dare Library
  DrRes_FrontHallPosi : DareLib/Dare/getAPI_type  g_funcname=Cdd_GetCurrentHallCnt  g_param=EN_DriverFront  g_type=uint16  g_size=-1
      settings: AttributesFormatString=%<g_funcname>  SourceProductName=Dare Library
  DrRes_FrontLockFault : DareLib/Dare/getAPI_type  g_funcname=Rte_GetVfb_DrFrontStallErr  g_param=""  g_type=uint8  g_size=-1
      settings: AttributesFormatString=%<g_funcname>  SourceProductName=Dare Library
  DrRes_HeightAutoRunFlag : DareLib/Dare/getAPI_type  g_funcname=Rte_GetVfb_DrHeightAutoRunFlag  g_param=""  g_type=uint8  g_enum=enSeatAutoRunSts  g_size=-1
      settings: AttributesFormatString=%<g_funcname>  SourceProductName=Dare Library
  DrRes_HeightDefaultMotorSize : DareLib/Dare/getAPI_type  g_funcname=Cdd_GetMotorSize  g_param=EN_DriverHeight  g_type=uint16  g_size=-1
      settings: AttributesFormatString=%<g_funcname>  SourceProductName=Dare Library
  DrRes_HeightDefaultStopPos : DareLib/Dare/getAPI_type  g_funcname=Cdd_GetMotorHardStop  g_param=EN_DriverHeight  g_type=uint16  g_size=-1
      settings: AttributesFormatString=%<g_funcname>  SourceProductName=Dare Library
  DrRes_HeightHallPosi : DareLib/Dare/getAPI_type  g_funcname=Cdd_GetCurrentHallCnt  g_param=EN_DriverHeight  g_type=uint16  g_size=-1
      settings: AttributesFormatString=%<g_funcname>  SourceProductName=Dare Library
  DrRes_HeightLockFault : DareLib/Dare/getAPI_type  g_funcname=Rte_GetVfb_DrHeightStallErr  g_param=""  g_type=uint8  g_size=-1
      settings: AttributesFormatString=%<g_funcname>  SourceProductName=Dare Library
  DrRes_IVI_NapMode_SwtichSet : DareLib/Dare/getAPI_type  g_funcname=CanRx_0x367_IVI_NapMode_SwtichSet  g_param=""  g_type=uint8  g_size=-1
      settings: AttributesFormatString=%<g_funcname>  SourceProductName=Dare Library
  DrRes_LengthAutoRunFlag : DareLib/Dare/getAPI_type  g_funcname=Rte_GetVfb_DrLengthAutoRunFlag  g_param=""  g_type=uint8  g_enum=enSeatAutoRunSts  g_size=-1
      settings: AttributesFormatString=%<g_funcname>  SourceProductName=Dare Library
  DrRes_LengthDefaultMotorSize : DareLib/Dare/getAPI_type  g_funcname=Cdd_GetMotorSize  g_param=EN_DriverLength  g_type=uint16  g_size=-1
      settings: AttributesFormatString=%<g_funcname>  SourceProductName=Dare Library
  DrRes_LengthDefaultStopPos : DareLib/Dare/getAPI_type  g_funcname=Cdd_GetMotorHardStop  g_param=EN_DriverLength  g_type=uint16  g_size=-1
      settings: AttributesFormatString=%<g_funcname>  SourceProductName=Dare Library
  DrRes_LengthHallPosi : DareLib/Dare/getAPI_type  g_funcname=Cdd_GetCurrentHallCnt  g_param=EN_DriverLength  g_type=uint16  g_size=-1
      settings: AttributesFormatString=%<g_funcname>  SourceProductName=Dare Library
  DrRes_LengthLockFault : DareLib/Dare/getAPI_type  g_funcname=Rte_GetVfb_DrLengthStallErr  g_param=""  g_type=uint8  g_size=-1
      settings: AttributesFormatString=%<g_funcname>  SourceProductName=Dare Library
  DrRes_MassageMode_FB : DareLib/Dare/getAPI_type  g_funcname=LinSignalGet_Massage_1_Massage_ModeSts_FB  g_param=""  g_type=uint8  g_enum=enMassageMode_DSM  g_size=-1
      settings: AttributesFormatString=%<g_funcname>  SourceProductName=Dare Library
  DrRes_PowerMode : DareLib/Dare/getAPI_type  g_funcname=Rte_GetVfb_PowerMode  g_param=""  g_type=uint8  g_enum=enPowerModeSts  g_size=-1
      settings: AttributesFormatString=%<g_funcname>  SourceProductName=Dare Library
  DrRes_SeatLearnResult : DareLib/Dare/getAPI_type  g_funcname=Rte_GetVfb_DrLearnResult  g_param=""  g_type=uint8  g_size=-1
      settings: AttributesFormatString=%<g_funcname>  SourceProductName=Dare Library
  DrRes_SeatMassageCfg : DareLib/Dare/getAPI_type  g_funcname=Srvl_GetMemIndexDataU8  g_param=EN_MemIndex_MassageConfig  g_type=uint8  g_size=-1
      settings: AttributesFormatString=%<g_funcname>  SourceProductName=Dare Library
  DrRes_VehicleRunFlag : DareLib/Dare/getAPI_type  g_funcname=Rte_GetVfb_VehicleRunFlag  g_param=""  g_type=uint8  g_size=-1
      settings: AttributesFormatString=%<g_funcname>  SourceProductName=Dare Library
  DrRes_VoltMode : DareLib/Dare/getAPI_type  g_funcname=Rte_GetVfb_VoltMode  g_param=""  g_type=uint8  g_enum=enFinalPowerMode  g_size=-1
      settings: AttributesFormatString=%<g_funcname>  SourceProductName=Dare Library
  DrRes_VoltSatisfy : DareLib/Dare/getAPI_type  g_funcname=Rte_GetVfb_VoltSatisfy  g_param=""  g_type=uint8  g_size=-1
      settings: AttributesFormatString=%<g_funcname>  SourceProductName=Dare Library
  DrRes_WelcomeEnable : DareLib/Dare/getAPI_type  g_funcname=Srvl_GetMemIndexDataU8  g_param=EN_MemIndex_DrMemoryConfig  g_type=uint8  g_size=-1
      settings: AttributesFormatString=%<g_funcname>  SourceProductName=Dare Library
  DrResl_ReCallPosi_Back : DareLib/Dare/getAPI_type  g_funcname=Srvl_GetMemIndexDataU16  g_param=EN_MemIndex_DrRes_ReCallPosi_Back  g_type=uint16  g_size=-1
      settings: AttributesFormatString=%<g_funcname>  SourceProductName=Dare Library
  DrResl_ReCallPosi_Front : DareLib/Dare/getAPI_type  g_funcname=Srvl_GetMemIndexDataU16  g_param=EN_MemIndex_DrRes_ReCallPosi_Front  g_type=uint16  g_size=-1
      settings: AttributesFormatString=%<g_funcname>  SourceProductName=Dare Library
  DrResl_ReCallPosi_Height : DareLib/Dare/getAPI_type  g_funcname=Srvl_GetMemIndexDataU16  g_param=EN_MemIndex_DrRes_ReCallPosi_Height  g_type=uint16  g_size=-1
      settings: AttributesFormatString=%<g_funcname>  SourceProductName=Dare Library
  DrResl_ReCallPosi_Length : DareLib/Dare/getAPI_type  g_funcname=Srvl_GetMemIndexDataU16  g_param=EN_MemIndex_DrRes_ReCallPosi_Length  g_type=uint16  g_size=-1
      settings: AttributesFormatString=%<g_funcname>  SourceProductName=Dare Library
  RTE_Signal : Outport
  wires:
  Bus Creator/1 -> RTE_Signal/1  "RTE_Signal"
  DrRes_HeightAutoRunFlag/1 -> Bus Creator/1  "DrRes_HeightAutoRunFlag"
  DrRes_LengthAutoRunFlag/1 -> Bus Creator/2  "DrRes_LengthAutoRunFlag"
  DrRes_BackAutoRunFlag/1 -> Bus Creator/3  "DrRes_BackAutoRunFlag"
  DrRes_FrontAutoRunFlag/1 -> Bus Creator/4  "DrRes_FrontAutoRunFlag"
  DrRes_HeightLockFault/1 -> Bus Creator/5  "DrRes_HeightLockFault"
  DrRes_LengthLockFault/1 -> Bus Creator/6  "DrRes_LengthLockFault"
  DrRes_BackLockFault/1 -> Bus Creator/7  "DrRes_BackLockFault"
  DrRes_FrontLockFault/1 -> Bus Creator/8  "DrRes_FrontLockFault"
  DrRes_DescHeightHallFault/1 -> Bus Creator/9  "DrRes_DescHeightHallFault"
  DrRes_DescLengthHallFault/1 -> Bus Creator/10  "DrRes_DescLengthHallFault"
  DrRes_DescBackHallFault/1 -> Bus Creator/11  "DrRes_DescBackHallFault"
  DrRes_DescFrontHallFault/1 -> Bus Creator/12  "DrRes_DescFrontHallFault"
  DrRes_AnyoneHallFaultSts/1 -> Bus Creator/13  "DrRes_AnyoneHallFaultSts"
  DrRes_AnyoneRelayFaultSts/1 -> Bus Creator/14  "DrRes_AnyoneRelayFaultSts"
  DrRes_CurrentMoveType/1 -> Bus Creator/15  "DrRes_CurrentMoveType"
  DrRes_SeatLearnResult/1 -> Bus Creator/16  "DrRes_SeatLearnResult"
  DrRes_VehicleRunFlag/1 -> Bus Creator/17  "DrRes_VehicleRunFlag"
  DrRes_EngineRunFlag/1 -> Bus Creator/18  "DrRes_EngineRunFlag"
  DrRes_HeightDefaultMotorSize/1 -> Bus Creator/19  "DrRes_HeightDefaultMotorSize"
  DrRes_LengthDefaultMotorSize/1 -> Bus Creator/20  "DrRes_LengthDefaultMotorSize"
  DrRes_BackDefaultMotorSize/1 -> Bus Creator/21  "DrRes_BackDefaultMotorSize"
  DrRes_FrontDefaulMotorSize/1 -> Bus Creator/22  "DrRes_FrontDefaulMotorSize"
  DrRes_HeightDefaultStopPos/1 -> Bus Creator/23  "DrRes_HeightDefaultStopPos"
  DrRes_LengthDefaultStopPos/1 -> Bus Creator/24  "DrRes_LengthDefaultStopPos"
  DrRes_BackDefaultStopPos/1 -> Bus Creator/25  "DrRes_BackDefaultStopPos"
  DrRes_FrontDefaulStoptPos/1 -> Bus Creator/26  "DrRes_FrontDefaulStoptPos"
  DrRes_HeightHallPosi/1 -> Bus Creator/27  "DrRes_HeightHallPosi"
  DrRes_LengthHallPosi/1 -> Bus Creator/28  "DrRes_LengthHallPosi"
  DrRes_BackHallPosi/1 -> Bus Creator/29  "DrRes_BackHallPosi"
  DrRes_FrontHallPosi/1 -> Bus Creator/30  "DrRes_FrontHallPosi"
  DrResl_ReCallPosi_Height/1 -> Bus Creator/31  "DrResl_ReCallPosi_Height"
  DrResl_ReCallPosi_Length/1 -> Bus Creator/32  "DrResl_ReCallPosi_Length"
  DrResl_ReCallPosi_Back/1 -> Bus Creator/33  "DrResl_ReCallPosi_Back"
  DrResl_ReCallPosi_Front/1 -> Bus Creator/34  "DrResl_ReCallPosi_Front"
  DrRes_AdjustEnable/1 -> Bus Creator/35  "DrRes_AdjustEnable"
  DrRes_WelcomeEnable/1 -> Bus Creator/36  "DrRes_WelcomeEnable"
  DrRes_SeatMassageCfg/1 -> Bus Creator/37  "DrRes_SeatMassageCfg"
  DrRes_MassageMode_FB/1 -> Bus Creator/38  "DrRes_MassageMode_FB"
  DrRes_IVI_NapMode_SwtichSet/1 -> Bus Creator/39  "DrRes_IVI_NapMode_SwtichSet"
  DrRes_PowerMode/1 -> Bus Creator/40  "DrRes_PowerMode"
  DrRes_VoltMode/1 -> Bus Creator/41  "DrRes_VoltMode"
  DrRes_VoltSatisfy/1 -> Bus Creator/42  "DrRes_VoltSatisfy"

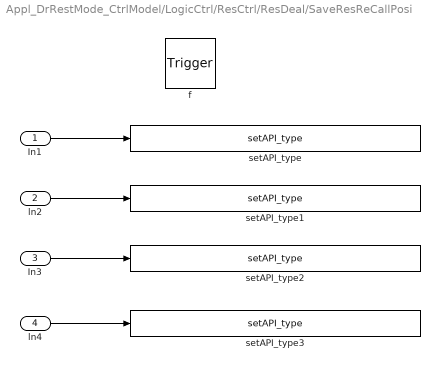
== system Appl_DrRestMode_CtrlModel/LogicCtrl/ResCtrl/ResDeal/SaveResReCallPosi ==
  In1 : Inport
  ln2 : Inport  Port=2
  In3 : Inport  Port=3
  ln4 : Inport  Port=4
  f : TriggerPort  TriggerType=function-call  VariantControl=(inherit)
      settings: CopyFcn=Stateflow.SLINSF.SimulinkMan.removeBlockPreDeleteFcn  PreDeleteFcn=Stateflow.SLINSF.SimulinkMan.unsafePredeleteFcn
  setAPI_type : DareLib/Dare/setAPI_type  g_funcname=Srvl_SetMemIndexDataU16  g_param=EN_MemIndex_DrRes_ReCallPosi_Height  g_type=uint16  g_size=-1
      settings: AttributesFormatString=%<g_funcname>  SourceProductName=Dare Library
  setAPI_type1 : DareLib/Dare/setAPI_type  g_funcname=Srvl_SetMemIndexDataU16  g_param=EN_MemIndex_DrRes_ReCallPosi_Length  g_type=uint16  g_size=-1
      settings: AttributesFormatString=%<g_funcname>  SourceProductName=Dare Library
  setAPI_type2 : DareLib/Dare/setAPI_type  g_funcname=Srvl_SetMemIndexDataU16  g_param=EN_MemIndex_DrRes_ReCallPosi_Back  g_type=uint16  g_size=-1
      settings: AttributesFormatString=%<g_funcname>  SourceProductName=Dare Library
  setAPI_type3 : DareLib/Dare/setAPI_type  g_funcname=Srvl_SetMemIndexDataU16  g_param=EN_MemIndex_DrRes_ReCallPosi_Front  g_type=uint16  g_size=-1
      settings: AttributesFormatString=%<g_funcname>  SourceProductName=Dare Library
  wires:
  In1/1 -> setAPI_type/1
  ln2/1 -> setAPI_type1/1
  In3/1 -> setAPI_type2/1
  ln4/1 -> setAPI_type3/1

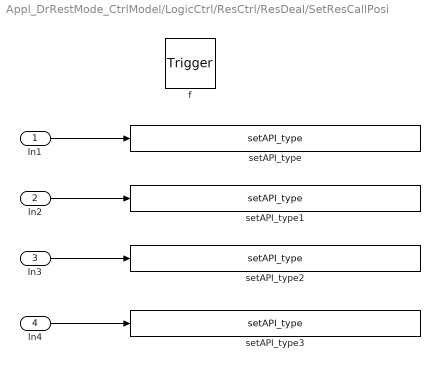
== system Appl_DrRestMode_CtrlModel/LogicCtrl/ResCtrl/ResDeal/SetResCallPosi ==
  In1 : Inport
  ln2 : Inport  Port=2
  In3 : Inport  Port=3
  ln4 : Inport  Port=4
  f : TriggerPort  TriggerType=function-call  VariantControl=(inherit)
      settings: CopyFcn=Stateflow.SLINSF.SimulinkMan.removeBlockPreDeleteFcn  PreDeleteFcn=Stateflow.SLINSF.SimulinkMan.unsafePredeleteFcn
  setAPI_type : DareLib/Dare/setAPI_type  g_funcname=Rte_SetVfb_Debug_Res_CallPosi_Height  g_param=""  g_type=uint16  g_size=-1
      settings: AttributesFormatString=%<g_funcname>  SourceProductName=Dare Library
  setAPI_type1 : DareLib/Dare/setAPI_type  g_funcname=Rte_SetVfb_Debug_Res_CallPosi_Length  g_param=""  g_type=uint16  g_size=-1
      settings: AttributesFormatString=%<g_funcname>  SourceProductName=Dare Library
  setAPI_type2 : DareLib/Dare/setAPI_type  g_funcname=Rte_SetVfb_Debug_Res_CallPosi_Back  g_param=""  g_type=uint16  g_size=-1
      settings: AttributesFormatString=%<g_funcname>  SourceProductName=Dare Library
  setAPI_type3 : DareLib/Dare/setAPI_type  g_funcname=Rte_SetVfb_Debug_Res_CallPosi_Front  g_param=""  g_type=uint16  g_size=-1
      settings: AttributesFormatString=%<g_funcname>  SourceProductName=Dare Library
  wires:
  In1/1 -> setAPI_type/1
  ln2/1 -> setAPI_type1/1
  In3/1 -> setAPI_type2/1
  ln4/1 -> setAPI_type3/1

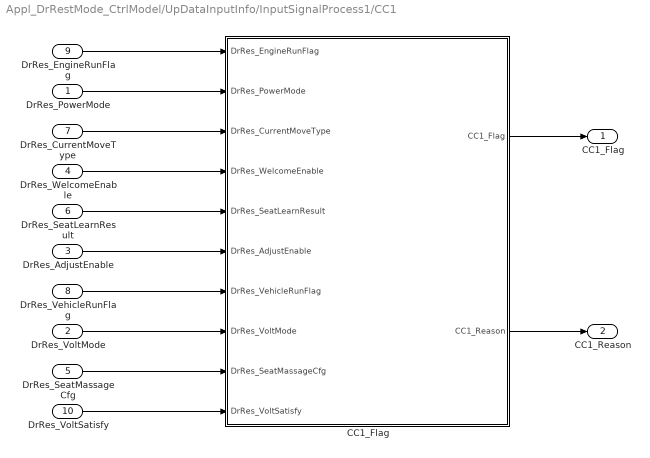
== system Appl_DrRestMode_CtrlModel/UpDataInputInfo/InputSignalProcess1/CC1 ==
  DrRes_PowerMode : Inport
  DrRes_VoltMode : Inport  Port=2
  DrRes_AdjustEnable : Inport  Port=3
  DrRes_WelcomeEnable : Inport  Port=4
  DrRes_SeatMassageCfg : Inport  Port=5
  DrRes_SeatLearnResult : Inport  Port=6
  DrRes_CurrentMoveType : Inport  Port=7
  DrRes_VehicleRunFlag : Inport  Port=8
  DrRes_EngineRunFlag : Inport  Port=9
  DrRes_VoltSatisfy : Inport  Port=10
  CC1_Flag : Stateflow chart  TreatAsAtomicUnit=on
  "CC1_Flag " : Outport
  CC1_Reason : Outport  Port=2
  wires:
  CC1_Flag/1(CC1_Flag) -> "CC1_Flag "/1
  CC1_Flag/2(CC1_Reason) -> CC1_Reason/1
  DrRes_EngineRunFlag/1 -> CC1_Flag/1(DrRes_EngineRunFlag)
  DrRes_PowerMode/1 -> CC1_Flag/2(DrRes_PowerMode)
  DrRes_CurrentMoveType/1 -> CC1_Flag/3(DrRes_CurrentMoveType)
  DrRes_WelcomeEnable/1 -> CC1_Flag/4(DrRes_WelcomeEnable)
  DrRes_SeatLearnResult/1 -> CC1_Flag/5(DrRes_SeatLearnResult)
  DrRes_AdjustEnable/1 -> CC1_Flag/6(DrRes_AdjustEnable)
  DrRes_VehicleRunFlag/1 -> CC1_Flag/7(DrRes_VehicleRunFlag)
  DrRes_VoltMode/1 -> CC1_Flag/8(DrRes_VoltMode)
  DrRes_SeatMassageCfg/1 -> CC1_Flag/9(DrRes_SeatMassageCfg)
  DrRes_VoltSatisfy/1 -> CC1_Flag/10(DrRes_VoltSatisfy)

== system Appl_DrRestMode_CtrlModel/UpDataInputInfo/InputSignalProcess1/CC2 ==
  DrRes_AdjustEnable : Inport
  DrRes_WelcomeEnable : Inport  Port=2
  DrRes_SeatLearnResult : Inport  Port=3
  CC2_Flag : Stateflow chart  TreatAsAtomicUnit=on
  "CC2_Flag " : Outport
  CC2_Reason : Outport  Port=2
  wires:
  CC2_Flag/2(CC2_Reason) -> CC2_Reason/1
  CC2_Flag/1(CC2_Flag) -> "CC2_Flag "/1
  DrRes_WelcomeEnable/1 -> CC2_Flag/3(DrRes_WelcomeEnable)
  DrRes_AdjustEnable/1 -> CC2_Flag/2(DrRes_AdjustEnable)
  DrRes_SeatLearnResult/1 -> CC2_Flag/1(DrRes_SeatLearnResult)

== system Appl_DrRestMode_CtrlModel/UpDataInputInfo/InputSignalProcess1/CC3 ==
  DrRes_SeatMassageCfg : Inport
  DrRes_PowerMode : Inport  Port=2
  DrRes_VehicleRunFlag : Inport  Port=3
  DrRes_EngineRunFlag : Inport  Port=4
  CC3_Flag : Stateflow chart  TreatAsAtomicUnit=on
  "CC3_Flag " : Outport
  CC3_Reason : Outport  Port=2
  wires:
  DrRes_PowerMode/1 -> CC3_Flag/1(DrRes_PowerMode)
  DrRes_SeatMassageCfg/1 -> CC3_Flag/3(DrRes_SeatMassageCfg)
  CC3_Flag/1(CC3_Flag) -> "CC3_Flag "/1
  CC3_Flag/2(CC3_Reason) -> CC3_Reason/1
  DrRes_EngineRunFlag/1 -> CC3_Flag/4(DrRes_EngineRunFlag)
  DrRes_VehicleRunFlag/1 -> CC3_Flag/2(DrRes_VehicleRunFlag)

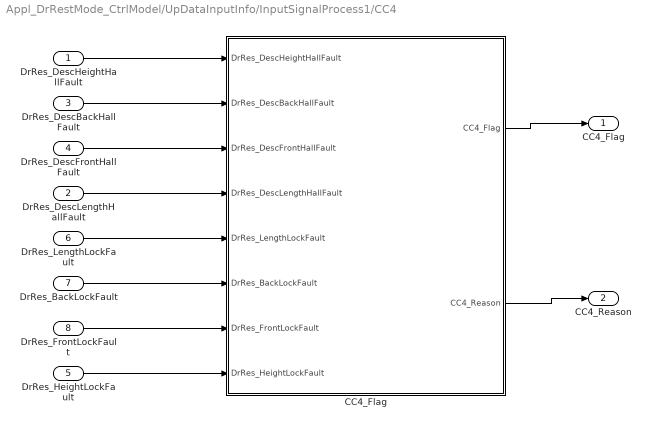
== system Appl_DrRestMode_CtrlModel/UpDataInputInfo/InputSignalProcess1/CC4 ==
  DrRes_DescHeightHallFault : Inport
  DrRes_DescLengthHallFault : Inport  Port=2
  DrRes_DescBackHallFault : Inport  Port=3
  DrRes_DescFrontHallFault : Inport  Port=4
  DrRes_HeightLockFault : Inport  Port=5
  DrRes_LengthLockFault : Inport  Port=6
  DrRes_BackLockFault : Inport  Port=7
  DrRes_FrontLockFault : Inport  Port=8
  CC4_Flag : Stateflow chart  TreatAsAtomicUnit=on
  "CC4_Flag " : Outport
  CC4_Reason : Outport  Port=2
  wires:
  DrRes_DescHeightHallFault/1 -> CC4_Flag/1(DrRes_DescHeightHallFault)
  CC4_Flag/1(CC4_Flag) -> "CC4_Flag "/1
  CC4_Flag/2(CC4_Reason) -> CC4_Reason/1
  DrRes_DescBackHallFault/1 -> CC4_Flag/2(DrRes_DescBackHallFault)
  DrRes_DescFrontHallFault/1 -> CC4_Flag/3(DrRes_DescFrontHallFault)
  DrRes_DescLengthHallFault/1 -> CC4_Flag/4(DrRes_DescLengthHallFault)
  DrRes_LengthLockFault/1 -> CC4_Flag/5(DrRes_LengthLockFault)
  DrRes_BackLockFault/1 -> CC4_Flag/6(DrRes_BackLockFault)
  DrRes_FrontLockFault/1 -> CC4_Flag/7(DrRes_FrontLockFault)
  DrRes_HeightLockFault/1 -> CC4_Flag/8(DrRes_HeightLockFault)

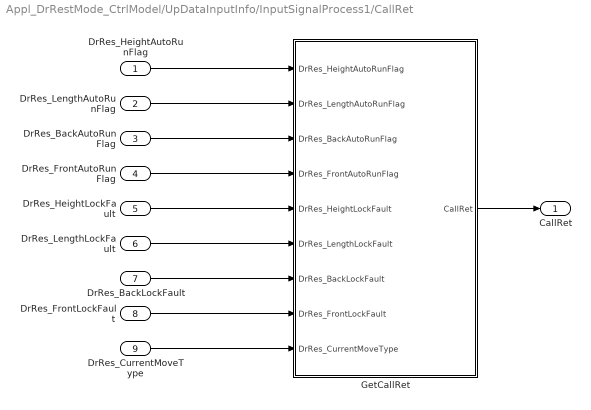
== system Appl_DrRestMode_CtrlModel/UpDataInputInfo/InputSignalProcess1/CallRet ==
  DrRes_HeightAutoRunFlag : Inport
  DrRes_LengthAutoRunFlag : Inport  Port=2
  DrRes_BackAutoRunFlag : Inport  Port=3
  DrRes_FrontAutoRunFlag : Inport  Port=4
  DrRes_HeightLockFault : Inport  Port=5
  DrRes_LengthLockFault : Inport  Port=6
  DrRes_BackLockFault : Inport  Port=7
  DrRes_FrontLockFault : Inport  Port=8
  DrRes_CurrentMoveType : Inport  Port=9
  GetCallRet : Stateflow chart  TreatAsAtomicUnit=on
  CallRet : Outport
  wires:
  GetCallRet/1(CallRet) -> CallRet/1
  DrRes_HeightAutoRunFlag/1 -> GetCallRet/1(DrRes_HeightAutoRunFlag)
  DrRes_LengthAutoRunFlag/1 -> GetCallRet/2(DrRes_LengthAutoRunFlag)
  DrRes_BackAutoRunFlag/1 -> GetCallRet/3(DrRes_BackAutoRunFlag)
  DrRes_FrontAutoRunFlag/1 -> GetCallRet/4(DrRes_FrontAutoRunFlag)
  DrRes_HeightLockFault/1 -> GetCallRet/5(DrRes_HeightLockFault)
  DrRes_LengthLockFault/1 -> GetCallRet/6(DrRes_LengthLockFault)
  DrRes_BackLockFault/1 -> GetCallRet/7(DrRes_BackLockFault)
  DrRes_FrontLockFault/1 -> GetCallRet/8(DrRes_FrontLockFault)
  DrRes_CurrentMoveType/1 -> GetCallRet/9(DrRes_CurrentMoveType)

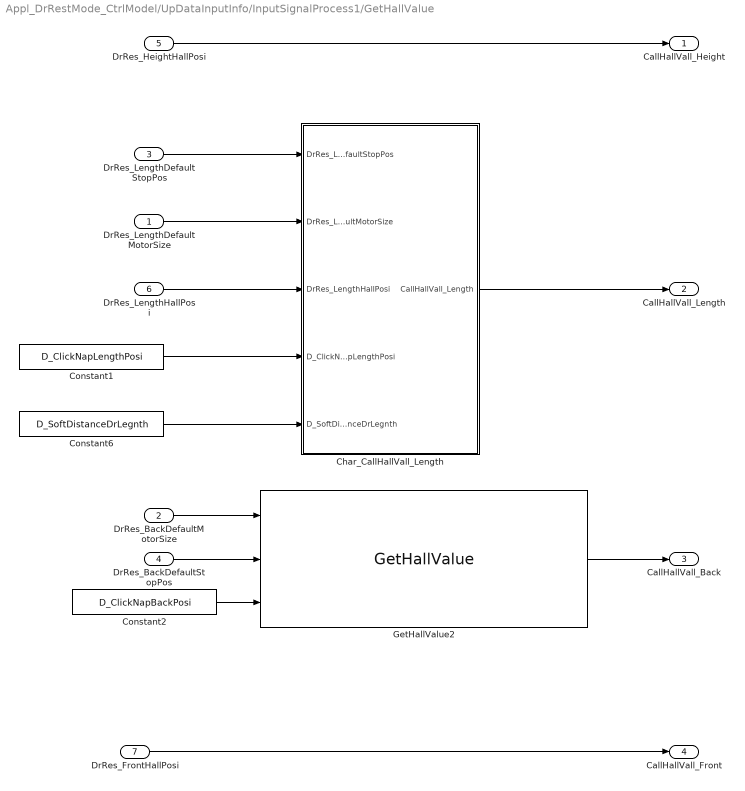
== system Appl_DrRestMode_CtrlModel/UpDataInputInfo/InputSignalProcess1/GetHallValue ==
  DrRes_LengthDefaultMotorSize : Inport
  DrRes_BackDefaultMotorSize : Inport  Port=2
  DrRes_LengthDefaultStopPos : Inport  Port=3
  DrRes_BackDefaultStopPos : Inport  Port=4
  DrRes_HeightHallPosi : Inport  Port=5
  DrRes_LengthHallPosi : Inport  Port=6
  DrRes_FrontHallPosi : Inport  Port=7
  Char_CallHallVall_Length : Stateflow chart  TreatAsAtomicUnit=on
  Constant1 : Constant  Value=D_ClickNapLengthPosi
  Constant2 : Constant  Value=D_ClickNapBackPosi
  Constant6 : Constant  Value=D_SoftDistanceDrLegnth
  GetHallValue2 : DareLib/Dare/GetHallValue  SystemSampleTime=-1
      settings: SourceProductName=Dare Library
  CallHallVall_Height : Outport  OutDataTypeStr=uint16
  CallHallVall_Length : Outport  Port=2  OutDataTypeStr=uint16
  CallHallVall_Back : Outport  Port=3  OutDataTypeStr=uint16
  CallHallVall_Front : Outport  Port=4  OutDataTypeStr=uint16
  wires:
  DrRes_BackDefaultMotorSize/1 -> GetHallValue2/1
  DrRes_BackDefaultStopPos/1 -> GetHallValue2/2
  Constant2/1 -> GetHallValue2/3
  Char_CallHallVall_Length/1(CallHallVall_Length) -> CallHallVall_Length/1
  GetHallValue2/1 -> CallHallVall_Back/1
  DrRes_HeightHallPosi/1 -> CallHallVall_Height/1
  DrRes_FrontHallPosi/1 -> CallHallVall_Front/1
  DrRes_LengthDefaultStopPos/1 -> Char_CallHallVall_Length/1(DrRes_LengthDefaultStopPos)
  DrRes_LengthDefaultMotorSize/1 -> Char_CallHallVall_Length/2(DrRes_LengthDefaultMotorSize)
  Constant1/1 -> Char_CallHallVall_Length/4(D_ClickNapLengthPosi)
  Constant6/1 -> Char_CallHallVall_Length/5(D_SoftDistanceDrLegnth)
  DrRes_LengthHallPosi/1 -> Char_CallHallVall_Length/3(DrRes_LengthHallPosi)

== system Appl_DrRestMode_CtrlModel/UpDataInputInfo/InputSignalProcess2/CLOSE ==
  DrRes_AnyoneRelayFaultSts : Inport
  DrRes_MassageMode_FB : Inport  Port=2
  DrRes_IVI_NapMode_SwtichSet : Inport  Port=3
  CC3_Flag : Inport  Port=4
  Colse_Flag : Stateflow chart  TreatAsAtomicUnit=on
  "Colse_Flag " : Outport
  Colse_Flag_Reason : Outport  Port=2
  wires:
  DrRes_IVI_NapMode_SwtichSet/1 -> Colse_Flag/2(DrRes_IVI_NapMode_SwtichSet)
  CC3_Flag/1 -> Colse_Flag/4(CC3_Flag)
  Colse_Flag/2(Close_Flag_Reason) -> Colse_Flag_Reason/1
  Colse_Flag/1(Close_Flag) -> "Colse_Flag "/1
  DrRes_AnyoneRelayFaultSts/1 -> Colse_Flag/3(DrRes_AnyoneRelayFaultSts)
  DrRes_MassageMode_FB/1 -> Colse_Flag/1(DrRes_MassageMode_FB)

== system Appl_DrRestMode_CtrlModel/UpDataInputInfo/InputSignalProcess2/GetDrRestCAllRet ==
  CallRet : Inport
  DrRestCAllRet : Outport
  wires:
  CallRet/1 -> DrRestCAllRet/1

== system Appl_DrRestMode_CtrlModel/UpDataInputInfo/InputSignalProcess2/MassageFault ==
  DrRes_MassageMode_FB : Inport
  MassageFault_Flag : Stateflow chart  TreatAsAtomicUnit=on
  "MassageFault_Flag " : Outport
  wires:
  DrRes_MassageMode_FB/1 -> MassageFault_Flag/1(DrRes_MassageMode_FB)
  MassageFault_Flag/1(MassageFault_Flag) -> "MassageFault_Flag "/1
